simulink library "components"  (R2018a)
settings: Solver=VariableStepAuto  StartTime=0.0  StopTime=10.0  RelTol=1e-3
libraries: fl_lib x9, nesl_utility x2
settings Model: Creator=Eric  LastModifiedBy=poker
settings DebuggingCC: LibraryContextMissingDiagnostic=warning
settings CodeAppCC: StateflowObjectComments=on

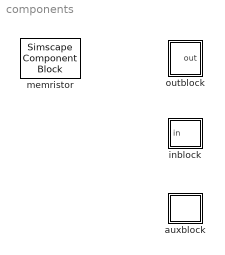
== system components ==
  auxblock : Subsystem
  inblock : Subsystem
  memristor : SimscapeComponentBlock  SourceFile=Memristor_ideal.Memristor_ideal  ComponentPath=Memristor_ideal.Memristor_ideal  ComponentVariants=Memristor_ideal.Memristor_ideal  ComponentVariantNames=Memristor_ideal  ClassName=Memristor_ideal  SchemaVersion=1  G1=0.9999 S  G0=0.0001 S  v_off=1 V  v_on=-1 V  w0=0  c1=1 V  c2=9.999e-6 s*V  w_specify=off  w_priority=None  w=0  w_nominal_specify=off  w_nominal_unit=1  w_nominal_value=1  i_specify=off  i_priority=None  i=0 A  i_nominal_specify=off  i_nominal_unit=A  i_nominal_value=1  v_specify=off  v_priority=None  v=0 V  v_nominal_specify=off  v_nominal_unit=V  v_nominal_value=1  power_dissipated_specify=off  power_dissipated_priority=None  power_dissipated=0 W  power_dissipated_nominal_specify=off  power_dissipated_nominal_unit=W  power_dissipated_nominal_value=1  mask(memristor){}
      settings: CopyFcn=simscape.engine.sli.internal.componentblockcallback(gcbh,'COPY')  PreCopyFcn=simscape.engine.sli.internal.componentblockcallback(gcbh,'PRECOPY')  PreDeleteFcn=simscape.engine.sli.internal.componentblockcallback(gcbh,'PREDELETE')
  outblock : Subsystem

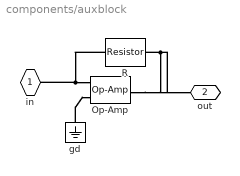
== system components/auxblock ==
  Op-Amp : fl_lib/Electrical/Electrical Elements/Op-Amp  outI_specify=off  outI_priority=None  outI=0 A  outI_nominal_specify=off  outI_nominal_unit=A  outI_nominal_value=1
  R : fl_lib/Electrical/Electrical Elements/Resistor  R=2 Ohm  i_specify=off  i_priority=None  i=0 A  i_nominal_specify=off  i_nominal_unit=A  i_nominal_value=1  v_specify=off  v_priority=None  v=0 V  v_nominal_specify=off  v_nominal_unit=V  v_nominal_value=1
  gd : fl_lib/Electrical/Electrical Elements/Electrical Reference
  in : PMIOPort  Side=Left
  out : PMIOPort  Port=2  Side=Right
  connections:
  R/LConn1 -- in/RConn1 -- Op-Amp/LConn2
  R/RConn1 -- out/RConn1 -- Op-Amp/RConn1
  gd/LConn1 -- Op-Amp/LConn1

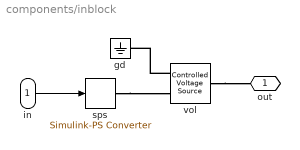
== system components/inblock ==
  in : Inport
  gd : fl_lib/Electrical/Electrical Elements/Electrical Reference
  sps : nesl_utility/Simulink-PS Converter  PhysicalDomain=network_engine_domain  SubClassName=ps_input  LeftPortType=input  RightPortType=output  PseudoPeriodic=off  Frequencies=[]  NoiseDistribution=none  NoiseParameters=[]  Unit=1  AffineConversion=off  FilteringAndDerivatives=zero  SimscapeFilterOrder=1  InputFilterTimeConstant=.001  UdotUserProvided=1
  vol : fl_lib/Electrical/Electrical Sources/Controlled Voltage Source
  out : PMIOPort  Side=Right
  wires:
  in/1 -> sps/1
  connections:
  sps/RConn1 -- vol/RConn1
  vol/RConn2 -- gd/LConn1
  vol/LConn1 -- out/RConn1

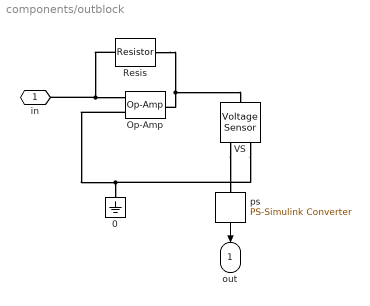
== system components/outblock ==
  0 : fl_lib/Electrical/Electrical Elements/Electrical Reference
  Op-Amp : fl_lib/Electrical/Electrical Elements/Op-Amp  outI_specify=off  outI_priority=None  outI=0 A  outI_nominal_specify=off  outI_nominal_unit=A  outI_nominal_value=1
  Resis : fl_lib/Electrical/Electrical Elements/Resistor  R=10 Ohm  i_specify=off  i_priority=None  i=0 A  i_nominal_specify=off  i_nominal_unit=A  i_nominal_value=1  v_specify=off  v_priority=None  v=0 V  v_nominal_specify=off  v_nominal_unit=V  v_nominal_value=1
  VS : fl_lib/Electrical/Electrical Sensors/Voltage Sensor
  ps : nesl_utility/PS-Simulink Converter  PhysicalDomain=network_engine_domain  SubClassName=ps_output  LeftPortType=input  RightPortType=output  PseudoPeriodic=off  Frequencies=[]  Unit=1  AffineConversion=off
  in : PMIOPort  Side=Left
  out : Outport
  wires:
  ps/1 -> out/1
  connections:
  Op-Amp/LConn1 -- VS/RConn2 -- 0/LConn1
  Resis/LConn1 -- in/RConn1 -- Op-Amp/LConn2
  Resis/RConn1 -- Op-Amp/RConn1 -- VS/LConn1
  VS/RConn1 -- ps/LConn1
